simulink model "kalman_estimate"  (R2018b)
settings: Solver=FixedStepAuto  StartTime=0.0  StopTime=2000  FixedStep=0.02  RelTol=1e-3
values from neighbouring files (symbols this model uses):
  D = randn(num_output,num_control)    [Com_of_linear_model_calculate.m]    (also in Copy_of_linear_model_calculate.m; D.mat = [0 0 0.00507528406191 0.0236369284061 0.221173094143 0.00198; LINEAR.m = randn(8,1)*10; MM_HKF.m = reshape(out(A_l+B_l+C_l+1:A_l+B_l+C_l+D_l),size_D))
  R = 0.003*eye(size(C,1))    [Com_of_kalman_gain.m]    (also in Copy_of_kalman_gain.m = diag(y_noise.^2); MM_HKF.m = diag(y_svar.^2); MM_based.m = diag(y_svar.^2); act_fault_of_kalman_gain.m = 0.02^2*eye(size(C,1)))
undefined symbols (not defined in the file or in its folder): Discrete, piece, Time
libraries: sharedschedule x16, commchan3 x1, ctrlSharedLib x1
settings Model: Creator=mmm  LastModifiedBy=mmm

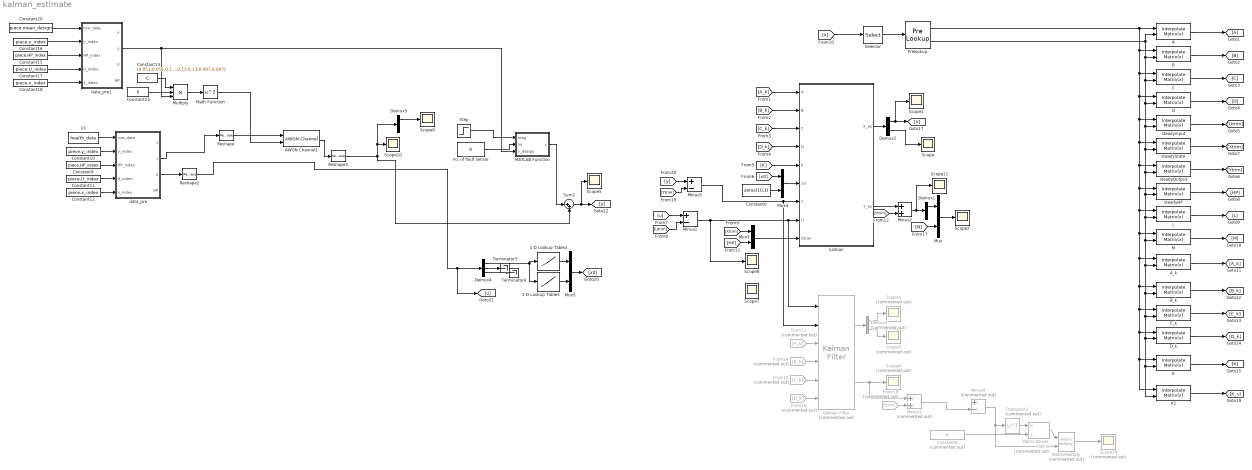
== system kalman_estimate ==
  1-D Lookup Table2 : Lookup_n-D  NumberOfTableDimensions=1  BreakpointsForDimension1=piece.u_stable_(:,1)  Table=piece.Nl  InterpMethod=Cubic spline  ExtrapMethod=Cubic spline  InternalRulePriority=Speed  RndMeth=Simplest  InputSameDT=on
  1-D Lookup Table3 : Lookup_n-D  NumberOfTableDimensions=1  BreakpointsForDimension1=piece.u_stable_(:,1)  Table=piece.x_stable_(:,2)  InterpMethod=Cubic spline  ExtrapMethod=Cubic spline  InternalRulePriority=Speed  RndMeth=Simplest  InputSameDT=on
  A : sharedschedule/Interpolate Matrix(x)   matrix=piece.A  aMode=aMode
      settings: SourceProductName=Aerospace Blockset  SourceProductBaseCode=AE
  AWGN Channel1 : commchan3/AWGN Channel  InputProcessing=Columns as channels (frame based)  seed=11:20  noiseMode=Variance from port  EbNodB=10  EsNodB=10  SNRdB=10  bitsPerSym=1  Ps=1  Tsym=1  variance=[2.55,7.5,0.03,0.03,0.3,0.3,0.15,0.15,0.45,0.45].^2
  A_k : sharedschedule/Interpolate Matrix(x)   matrix=piece.A_k  aMode=aMode
      settings: SourceProductName=Aerospace Blockset  SourceProductBaseCode=AE
  B : sharedschedule/Interpolate Matrix(x)   matrix=piece.B  aMode=aMode
      settings: SourceProductName=Aerospace Blockset  SourceProductBaseCode=AE
  B_k : sharedschedule/Interpolate Matrix(x)   matrix=piece.B_k  aMode=aMode
      settings: SourceProductName=Aerospace Blockset  SourceProductBaseCode=AE
  C : sharedschedule/Interpolate Matrix(x)   matrix=piece.C  aMode=aMode
      settings: SourceProductName=Aerospace Blockset  SourceProductBaseCode=AE
  C_k : sharedschedule/Interpolate Matrix(x)   matrix=piece.C_k  aMode=aMode
      settings: SourceProductName=Aerospace Blockset  SourceProductBaseCode=AE
  Constant10 : Constant  Value=piece.y_index
  Constant11 : Constant  Value=piece.U_index
  Constant12 : Constant  Value=piece.x_index
  Constant13 : Constant  Value=[0.051,0.051,0.164,0.164,0.15,0.15,0.13,0.13,0.097,0.097]  VectorParams1D=off
  Constant14 : Constant  Value=0
  Constant15 : Constant  Value=piece.HP_index
  Constant16 : Constant  Value=piece.y_index
  Constant17 : Constant  Value=piece.U_index
  Constant18 : Constant  Value=piece.x_index
  Constant20 : Constant  Value=piece.mean_design  VectorParams1D=off
  Constant6 : Constant  Value=zeros(10,1)  VectorParams1D=off
  Constant8 : Constant  Commented=on  Value=R  VectorParams1D=off
  Constant9 : Constant  Value=piece.HP_index
  D : sharedschedule/Interpolate Matrix(x)   matrix=piece.D  aMode=aMode
      settings: SourceProductName=Aerospace Blockset  SourceProductBaseCode=AE
  D_k : sharedschedule/Interpolate Matrix(x)   matrix=piece.D_k  aMode=aMode
      settings: SourceProductName=Aerospace Blockset  SourceProductBaseCode=AE
  Demux1 : Demux  Outputs=[1,1,8]
  Demux2 : Demux  Outputs=[2,10]
  Demux3 : Demux  Commented=on  Outputs=[2,10]
  Demux4 : Demux  Outputs=3
  Demux5 : Demux  Outputs=[1,9]
  From13 : From  Commented=on  GotoTag=A_k
  From14 : From  Commented=on  GotoTag=B_k
  From15 : From  Commented=on  GotoTag=C_k
  From16 : From  Commented=on  GotoTag=D_k
  From18 : From  Commented=on  GotoTag=Ytrim
  K : sharedschedule/Interpolate Matrix(x)   matrix=piece.K  aMode=aMode
      settings: SourceProductName=Aerospace Blockset  SourceProductBaseCode=AE
  K1 : sharedschedule/Interpolate Matrix(x)   matrix=piece.K_s  aMode=aMode
      settings: SourceProductName=Aerospace Blockset  SourceProductBaseCode=AE
  Kalman Filter : ctrlSharedLib/Kalman Filter  Commented=on  TimeDomain=Discrete-Time  UseCurrentEstimator=on  ModelSource=Input port  ModelSourceVariable=ss(0.95,1,1,0,1)  A=0.95  B=1  C=1  D=0  NumberOfStates=12  NumberOfInputs=3  NumberOfOutputs=10  InitialEstimateSource=Dialog  X0=0  P0=10  UseK=off  UseGH=off  NumberOfProcessNoiseInputs=1  G=1  TimeInvariantG=on  H=0  TimeInvariantH=on  Q=0.02^2  TimeInvariantQ=on  R=1  TimeInvariantR=on  N=0  TimeInvariantN=on  AddInputPort=on  AddEnablePort=off  OutputEstimatedY=on  OutputP=off  Ts=-1
      settings: SourceProductBaseCode=CT
  L : sharedschedule/Interpolate Matrix(x)   matrix=piece.L  aMode=aMode
      settings: SourceProductName=Aerospace Blockset  SourceProductBaseCode=AE
  M : sharedschedule/Interpolate Matrix(x)   matrix=piece.M  aMode=aMode
      settings: SourceProductName=Aerospace Blockset  SourceProductBaseCode=AE
  MATLAB Function : MATLAB Function  TreatAsAtomicUnit=on
  Math Function : Math  Operator=square  SaturateOnIntegerOverflow=on
  Matrix Divide : Product  Commented=on  Inputs=*/  Multiplication=Matrix(*)
  MatrixMultiply : Product  Commented=on  Multiplication=Matrix(*)
  Minus1 : Sum  Inputs=+-
  Minus2 : Sum
  Minus3 : Sum  Commented=on
  Minus4 : Sum  Commented=on  Inputs=+-
  Minus5 : Sum  Inputs=+-
  Multiply : Product  Inputs=3
  Mux{,3..5} (4 alike) : Mux  Inputs=2
  Prelookup : PreLookup  BreakpointsData=piece.Nl  BreakpointObject=Nl  ExtrapMethod=Linear  UseLastBreakpoint=on  DiagnosticForOutOfRangeInput=Warning
  Reshape : Reshape  OutputDimensionality=Row vector (2-D)
  Reshape2 : Reshape  OutputDimensionality=Column vector (2-D)
  Reshape3 : Reshape  OutputDimensionality=Column vector (2-D)
  Scope{,1..2,5,7..11} (9 alike) : Scope
  Scope{3..4,6,19} (4 alike) : Scope  Commented=on
  Selector : Selector  InputPortWidth=2  IndexOptions=Index vector (dialog)  Indices=[1]  OutputSizes=1
  Step : Step  Time=50  After=-0.02  SampleTime=0
  Sum2 : Sum  Inputs=|++
  Terminator3 : Terminator
  Terminator4 : Terminator
  Transpose2 : Math  Commented=on  Operator=transpose  SaturateOnIntegerOverflow=on
  U1 : FromWorkspace  VariableName=health_data  SampleTime=0.02  Interpolate=off  OutputAfterFinalValue=Holding final value
  data_pre : MATLAB Function  TreatAsAtomicUnit=on
  data_pre1 : MATLAB Function  TreatAsAtomicUnit=on
  "kalman " : Subsystem
  no. of fault sensor : Constant  Value=6
  steadyHP : sharedschedule/Interpolate Matrix(x)   matrix=piece.steadyHP  aMode=aMode
      settings: SourceProductName=Aerospace Blockset  SourceProductBaseCode=AE
  steadyOutput : sharedschedule/Interpolate Matrix(x)   matrix=piece.steadyOutput  aMode=aMode
      settings: SourceProductName=Aerospace Blockset  SourceProductBaseCode=AE
  steadyState : sharedschedule/Interpolate Matrix(x)   matrix=piece.steadyState  aMode=aMode
      settings: SourceProductName=Aerospace Blockset  SourceProductBaseCode=AE
  steadyinput : sharedschedule/Interpolate Matrix(x)   matrix=piece.steadyInput  aMode=aMode
      settings: SourceProductName=Aerospace Blockset  SourceProductBaseCode=AE
  wires:
  K/1 -> [K]
  B_k/1 -> [B_k]
  C_k/1 -> [C_k]
  D_k/1 -> [D_k]
  A_k/1 -> [A_k]
  steadyinput/1 -> [Utrim]
  [X] -> Selector/1
  Prelookup/2 -> A/2, steadyState/2, steadyOutput/2, steadyHP/2, L/2, B_k/2, C_k/2, K1/2, K/2, D_k/2, A_k/2, M/2, steadyinput/2, D/2, C/2, B/2
  steadyState/1 -> [Xtrim]
  B/1 -> [B]
  steadyHP/1 -> [HP]
  steadyOutput/1 -> [Ytrim]
  D/1 -> [D]
  A/1 -> [A]
  C/1 -> [C]
  L/1 -> [L]
  M/1 -> [M]
  Prelookup/1 -> steadyState/1, steadyOutput/1, steadyHP/1, L/1, B_k/1, C_k/1, K1/1, K/1, D_k/1, A_k/1, M/1, steadyinput/1, D/1, C/1, B/1, A/1
  Selector/1 -> Prelookup/1
  [A_k] -> "kalman "/1(A)
  [B_k] -> "kalman "/2(B)
  [C_k] -> "kalman "/3(C)
  [D_k] -> "kalman "/4(D)
  [K] -> "kalman "/5(K)
  [Utrim] -> Minus1/2
  [Xtrim] -> Mux3/1
  [HP] -> Mux3/2
  Mux3/1 -> "kalman "/9(Xtrim)
  "kalman "/1(X_es) -> Demux2/1
  Demux2/1 -> Scope1/1, [X]
  [x0] -> Mux4/1
  Constant6/1 -> Mux4/2
  Mux4/1 -> "kalman "/6(x0)
  "kalman "/2(Y_es) -> Minus2/1
  [Ytrim] -> Minus2/2
  Minus2/1 -> Scope11/1, Demux1/1
  From13/1 -> Kalman Filter/3
  From14/1 -> Kalman Filter/4
  From15/1 -> Kalman Filter/5
  From16/1 -> Kalman Filter/6
  Demux3/2 -> Scope3/1
  Demux3/1 -> Scope4/1
  Kalman Filter/1 -> Demux3/1
  Demux1/1 -> Mux/1
  [N] -> Mux/2
  Mux/1 -> Scope2/1
  Demux2/2 -> Scope/1
  Kalman Filter/2 -> Minus3/1, Scope6/1
  From18/1 -> Minus3/2
  Constant8/1 -> Matrix Divide/2
  Matrix Divide/1 -> MatrixMultiply/1
  MatrixMultiply/1 -> Scope19/1
  Transpose2/1 -> Matrix Divide/1
  Minus4/1 -> MatrixMultiply/2, Transpose2/1
  Minus3/1 -> Minus4/2
  K1/1 -> [K_s]
  Minus1/1 -> Scope8/1, Kalman Filter/1, "kalman "/8(U)
  Reshape2/1 -> [u], Demux4/1
  Demux4/1 -> 1-D Lookup Table3/1, 1-D Lookup Table2/1
  Constant18/1 -> data_pre1/5(x_index)
  Reshape3/1 -> Sum2/2, Scope10/1, Demux5/1
  Constant9/1 -> data_pre/3(HP_index)
  Demux5/1 -> Scope9/1
  data_pre/2(y) -> Reshape/1
  Reshape/1 -> AWGN Channel1/1
  data_pre1/2(y) -> Multiply/3, MATLAB Function/3(y_design)
  Constant16/1 -> data_pre1/2(y_index)
  data_pre/3(U) -> Reshape2/1
  Constant17/1 -> data_pre1/4(U_index)
  Constant15/1 -> data_pre1/3(HP_index)
  Constant12/1 -> data_pre/5(x_index)
  Constant11/1 -> data_pre/4(U_index)
  U1/1 -> data_pre/1(row_data)
  1-D Lookup Table2/1 -> Mux5/1
  no. of fault sensor/1 -> MATLAB Function/2(no)
  Step/1 -> MATLAB Function/1(mag)
  Constant10/1 -> data_pre/2(y_index)
  Mux5/1 -> [x0]
  1-D Lookup Table3/1 -> Mux5/2
  Constant13/1 -> Multiply/1
  Constant14/1 -> Multiply/2
  AWGN Channel1/1 -> Reshape3/1
  Sum2/1 -> Scope5/1, [y]
  Demux4/3 -> Terminator4/1
  Constant20/1 -> data_pre1/1(row_data)
  MATLAB Function/1(y) -> Sum2/1
  Math Function/1 -> AWGN Channel1/2
  Demux4/2 -> Terminator3/1
  Multiply/1 -> Math Function/1
  [u] -> Minus1/1
  [y] -> Minus5/1
  [Ytrim] -> Minus5/2
  Minus5/1 -> Kalman Filter/2, "kalman "/7(Y)

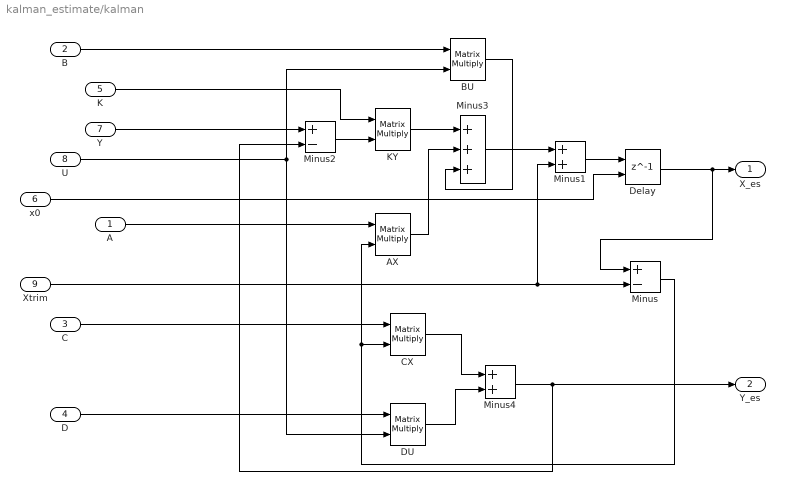
== system kalman_estimate/kalman  ==
  A : Inport
  B : Inport  Port=2
  C : Inport  Port=3
  D : Inport  Port=4
  K : Inport  Port=5
  x0 : Inport  Port=6
  Y : Inport  Port=7
  U : Inport  Port=8
  Xtrim : Inport  Port=9
  "\tCX" : Product  Multiplication=Matrix(*)
  AX : Product  Multiplication=Matrix(*)
  BU : Product  Multiplication=Matrix(*)
  DU : Product  Multiplication=Matrix(*)
  Delay : Delay  DelayLength=1  InitialConditionSource=Input port
      settings: InputPortMap=u0,p4
  KY : Product  Multiplication=Matrix(*)
  Minus : Sum  Inputs=+-
  Minus1 : Sum
  Minus2 : Sum  Inputs=+-
  Minus3 : Sum  Inputs=+++
  Minus4 : Sum
  X_es : Outport
  Y_es : Outport  Port=2
  wires:
  Minus4/1 -> Minus2/2, Y_es/1
  KY/1 -> Minus3/1
  U/1 -> BU/2, DU/2
  Y/1 -> Minus2/1
  DU/1 -> Minus4/2
  "\tCX"/1 -> Minus4/1
  x0/1 -> Delay/2
  Minus2/1 -> KY/2
  BU/1 -> Minus3/3
  A/1 -> AX/1
  B/1 -> BU/1
  C/1 -> "\tCX"/1
  D/1 -> DU/1
  K/1 -> KY/1
  Xtrim/1 -> Minus1/2, Minus/2
  Delay/1 -> Minus/1, X_es/1
  Minus/1 -> AX/2, "\tCX"/2
  AX/1 -> Minus3/2
  Minus3/1 -> Minus1/1
  Minus1/1 -> Delay/1

== matlab function kalman_estimate/data_pre ==
  data: x output; row_data input; y output; y_index input; HP_index input; U_index input; x_index input; U output; HP output
function[x,y,U,HP] = fcn(row_data,y_index,HP_index,U_index,x_index)
%%% 数据相似归一化
% if size(mean_design,1) > size(mean_design,2)
%     mean_ = mean_design';
% else
%     mean_ = mean_design;
% end
if size(y_index,1) > size(y_index,2)
    y_index_ = y_index';
else
    y_index_ =y_index;
end
if size(x_index,1) > size(x_index,2)
    x_index_ = x_index';
else
    x_index_ = x_index;   
end
if size(HP_index,1) > size(HP_index,2)
    HP_index_ = HP_index';
else
    HP_index_ = HP_index;
end
if size(U_index,1) > size(U_index,2)
    U_index_ = U_index';
else
    U_index_ = U_index;
end

if size(row_data,1)>size(row_data,2)
    row = row_data';
else
    row = row_data;
end

y = row(:,y_index_)';
x = row(:,x_index_)';
HP = row(:,HP_index_)'-1;
U = row(:,U_index_)';

== matlab function kalman_estimate/data_pre1 ==
  data: x output; row_data input; y output; y_index input; HP_index input; U_index input; x_index input; U output; HP output
function[x,y,U,HP] = fcn(row_data,y_index,HP_index,U_index,x_index)
%%% 数据相似归一化
% if size(mean_design,1) > size(mean_design,2)
%     mean_ = mean_design';
% else
%     mean_ = mean_design;
% end
if size(y_index,1) > size(y_index,2)
    y_index_ = y_index';
else
    y_index_ =y_index;
end
if size(x_index,1) > size(x_index,2)
    x_index_ = x_index';
else
    x_index_ = x_index;   
end
if size(HP_index,1) > size(HP_index,2)
    HP_index_ = HP_index';
else
    HP_index_ = HP_index;
end
if size(U_index,1) > size(U_index,2)
    U_index_ = U_index';
else
    U_index_ = U_index;
end

if size(row_data,1)>size(row_data,2)
    row = row_data';
else
    row = row_data;
end

y = row(:,y_index_)';
x = row(:,x_index_)';
HP = row(:,HP_index_)'-1;
U = row(:,U_index_)';

== matlab function kalman_estimate/MATLAB Function ==
  data: mag input; y output; no input; y_design input
function y = fcn(mag,no,y_design)
y_ = zeros(1,10);
y_(no) = mag*y_design(no);
y = y_';
end
